simulink model "finalserial"  (R2020a)
settings: Solver=VariableStepAuto  StartTime=0.0  StopTime=10.0  RelTol=1e-3
libraries: xpcutilitieslib x2
settings Model: Creator=JClae  LastModifiedBy=JClae

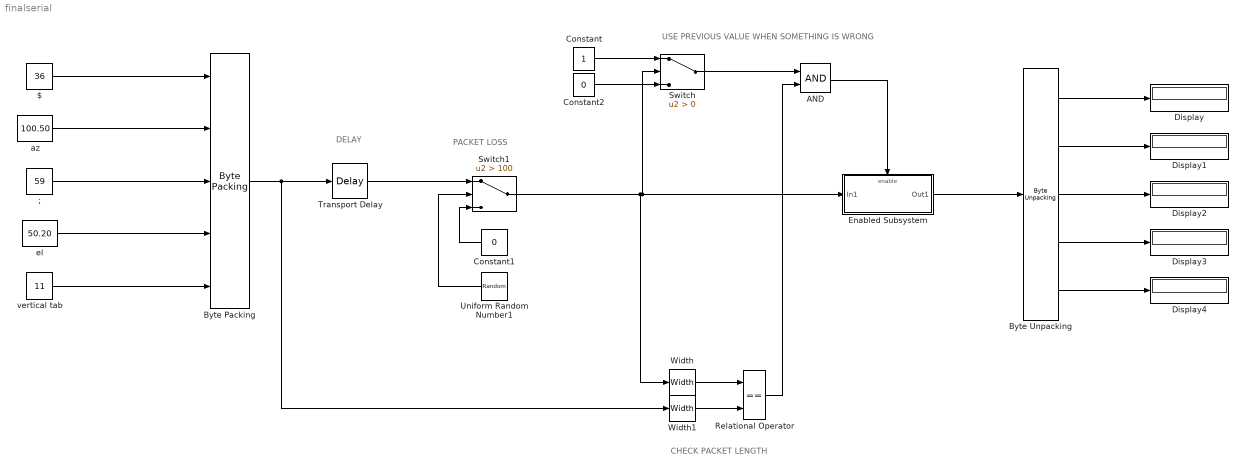
== system finalserial ==
  note: USE PREVIOUS VALUE WHEN SOMETHING IS WRONG
  note: CHECK PACKET LENGTH
  note: PACKET LOSS
  note: DELAY
  $ : Constant  Value=36  OutMin=0  OutMax=360  OutDataTypeStr=single
  ; : Constant  Value=59  OutMin=0  OutMax=255  OutDataTypeStr=single
  AND : Logic  AllPortsSameDT=off  OutDataTypeStr=boolean
  "Byte Packing " : xpcutilitieslib/Byte Packing   MaskPackedDataType=double  MaskUnpackedDataTypes={'single','double','single','double','single'}  MaskAlignment=1
  "Byte Unpacking " : xpcutilitieslib/Byte Unpacking   MaskUnpackedDataTypes={'single','double','single','double','single'}  MaskUnpackedDataSizes={[1],[1],[1],[1],[1]}  MaskAlignment=1
      settings: SourceProductBaseCode=XP
  Constant : Constant
  Constant1 : Constant  Value=0
  Constant2 : Constant  Value=0
  Display{,1..4} (5 alike) : Display
  Enabled Subsystem : Subsystem  TreatAsAtomicUnit=on
  Relational Operator : RelationalOperator  Operator===  OutDataTypeStr=boolean  RndMeth=Simplest
  Switch : Switch  Criteria=u2 > Threshold
  Switch1 : Switch  Criteria=u2 > Threshold  Threshold=100
  Transport Delay : TransportDelay  DelayTime=5
  Uniform Random Number1 : UniformRandomNumber  Minimum=0  Maximum=100  Seed=5  SampleTime=0.1
  Width : Width
  Width1 : Width
  az : Constant  Value=100.50  OutMin=0  OutMax=180  OutDataTypeStr=double
  el : Constant  Value=50.20  OutMin=0  OutMax=180  OutDataTypeStr=double
  vertical tab : Constant  Value=11  OutMin=0  OutMax=255  OutDataTypeStr=single
  wires:
  $/1 -> "Byte Packing "/1
  ;/1 -> "Byte Packing "/3
  "Byte Unpacking "/3 -> Display2/1
  "Byte Unpacking "/2 -> Display1/1
  vertical tab/1 -> "Byte Packing "/5
  az/1 -> "Byte Packing "/2
  el/1 -> "Byte Packing "/4
  "Byte Unpacking "/4 -> Display3/1
  "Byte Unpacking "/5 -> Display4/1
  "Byte Packing "/1 -> Transport Delay/1, Width1/1
  "Byte Unpacking "/1 -> Display/1
  Switch1/1 -> Width/1, Switch/2, Enabled Subsystem/1(In1)
  Constant1/1 -> Switch1/3
  Uniform Random Number1/1 -> Switch1/2
  Width/1 -> Relational Operator/1
  Width1/1 -> Relational Operator/2
  Transport Delay/1 -> Switch1/1
  Enabled Subsystem/1(Out1) -> "Byte Unpacking "/1
  Constant/1 -> Switch/1
  Constant2/1 -> Switch/3
  Relational Operator/1 -> AND/2
  Switch/1 -> AND/1
  AND/1 -> Enabled Subsystem/Enable

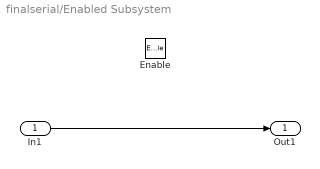
== system finalserial/Enabled Subsystem ==
  In1 : Inport
  Enable : EnablePort
  Out1 : Outport
  wires:
  In1/1 -> Out1/1
